simulink model "px4_control_system"  (R2023b)
settings: Solver=FixedStepAuto  StartTime=0.0  StopTime=inf  RelTol=1e-3  EnableMultiTasking=on
InitFcn:
  | prepare
values from neighbouring files (symbols this model uses):
  g = G_RPY18(x,p)    [CalculateLghn.m]
  m = 1    [CovarianceCheck.m]    (also in FL.m = in2(:,1); Fe1.m = in5(:,1); Fe1Fj.m = ct{4}; Fe1Gj.m = in5(:,1))
undefined symbols (not defined in the file or in its folder): AUX, color, dev, DiscIntNeverNeededParam, invC, J, led_mask, mode, pwm_output1
libraries: simulink x12, px4Sensorslib x4, px4uORBlib x2, px4lib x1
(part 2 of 2)

== matlab function px4_control_system/Subsystem/PX4 SD Card Logger1/SDCard_logger ==
  data: en input boolean; data input; logname parameter uint8; cacheflag parameter boolean; numRecs parameter uint32
%% PX4 SD Card Logger
% Note: All data needs to be of the same type (e.g. double)
% Header information format:
%           String "MWLOG"
%           Time/Date 4 bytes (time())
%           Number of Signals per record Logged 1 byte (256 max)
%           Data Type of Signals Logged  1 byte (1-10)
%           Number of bytes per record 2 bytes (65535 max)
% This does NOT include the number of data sets logged.
% i.e. The Reader is responsible for reading until EOF.
% Steve Kuznicki
% Copyright 2018 The MathWorks, Inc.

function SDCard_logger(en, data, logname, cacheflag, numRecs)

persistent fp isflushed isopen count  elem_size vect_size datastore timestore count_prev

if coder.target('Rtw')
    
    coder.cinclude('<stdio.h>');
    coder.cinclude('<time.h>');
    
    if coder.target('Rtw')
        coder.cinclude('<drivers/drv_hrt.h>');
    end
    
    if coder.target('Rtw')
        timestamp=coder.opaque('uint64_t');
        timestamp=coder.ceval('hrt_absolute_time');
    else
        timestamp = uint64(0);
    end
    
    if isempty(count)
        count = uint32(0);
        count_prev=count;
        fp = coder.opaque('FILE*', 'NULL');
        isflushed = false;
        if cacheflag == true
            datastore = zeros(numRecs*uint32(coder.const(numel(data))), 1, 'like', data);
            timestore=uint64(zeros(numRecs, 1));
        end
        
        [elsize, eltype] = get_elem_size(data);
        elem_size = coder.const(uint16(elsize));
        elem_type = coder.const(uint8(eltype));
        vect_size = coder.const(uint8(numel(data)));
        coder.ceval('printf',['OPENING file %s vect_size %d elem_size %d numRecs %d %c' uint8(0)], ...
            [logname,'.bin', int8(0)], uint32(vect_size), uint32(elem_size), uint32(numRecs), uint8(10));
        fp = coder.ceval('fopen', [logname,'.bin', int8(0)], ['wb', int8(0)]);
        isopen = true;
        
        % Write header information here
        % header token + version
        mlStrVer = 'MWLOG';
        coder.ceval('fwrite', coder.rref(mlStrVer), uint32(1), length(mlStrVer), fp);
        % date/time
        tm = uint32(0);
        tmptr = uint32(0);
        tm = coder.ceval('time',coder.wref(tmptr));
        coder.ceval('fwrite', coder.rref(tm), uint32(4), uint32(1), fp);
        % number of elements in each record
        coder.ceval('fwrite', coder.rref(vect_size), uint32(1), uint32(1), fp);
        % data type of the elements
        coder.ceval('fwrite', coder.rref(elem_type), uint32(1), uint32(1), fp);
        % size of each record in bytes
        recSize = elem_size * uint16(vect_size);
        coder.ceval('fwrite', coder.rref(recSize), uint32(2), uint32(1), fp);
    end
    
    
    if (en && (count < numRecs))
        
        if isopen == false
            % open file in append mode
            fp = coder.ceval('fopen', [logname,'.bin', int8(0)], ['ab', int8(0)]);
            isflushed = false;
            isopen = true;
            count_prev=count;
        end
        
        % cache data in memory or use fwrite
        if cacheflag == true
            addr = (count*uint32(vect_size))+1;
            for idx = 1:vect_size
                datastore(addr) = data(idx);
                addr = addr + 1;
            end
            timestore(count+uint32(1))=uint64(timestamp);
        else
            coder.ceval('fwrite', coder.rref(data), elem_size, vect_size, fp);
            if coder.target('Rtw')
                coder.ceval('fwrite', coder.rref(timestamp), uint32(8), uint32(1), fp);
            end
        end
        count = count + uint32(1);
        
    else
        if isopen == true
            if ~isflushed
                coder.ceval('printf',['CLOSING file. count = %d %c' uint8(0)], uint32(count), uint8(10));
                if cacheflag
                    for idx=count_prev+1:count
                        for idx2=(idx-1)*double(vect_size)+1:(idx-1)*double(vect_size)+double(vect_size)
                            coder.ceval('fwrite', coder.rref(datastore(idx2)), elem_size, uint32(1), fp);
                        end
                        coder.ceval('fwrite', coder.rref(timestore(idx)), uint32(8), uint32(1), fp);
                    end
                end
                coder.ceval('fflush', fp);
                isflushed = true;
            end
            coder.ceval('fclose', fp);
        end
        isopen = false;
    end
end

% return the size of the element in bytes
    function [elem_size, dtype] = get_elem_size(data)
        switch(class(data))
            case 'double'
                elem_size = 8;
                dtype = 1;
            case 'single'
                elem_size = 4;
                dtype = 2;
            case 'int32'
                elem_size = 4;
                dtype = 3;
            case 'uint32'
                elem_size = 4;
                dtype = 4;
            case 'int16'
                elem_size = 2;
                dtype = 5;
            case 'uint16'
                elem_size = 2;
                dtype = 6;
            case 'int8'
                elem_size = 1;
                dtype = 7;
            case 'uint8'
                elem_size = 1;
                dtype = 8;
            case 'logical'
                elem_size = 1;
                dtype = 9;
            case 'embedded.fi'
                nt = numerictype(data);
                elem_size = 2^ceil(log2(ceil(nt.WordLength / 8)));
                dtype = 10;
        end
        if ~isreal(data)
            elem_size = elem_size*2;
        end
        
        elem_size = uint16(elem_size);
        dtype = uint8(dtype);
    end
end

== matlab function px4_control_system/Control/MATLAB Function1 ==
  data: u input; y output
function y = ned2enu(u)
y = [u(2); u(1); -u(3)];

== matlab function px4_control_system/Subsystem/PX4 SD Card Logger2/SDCard_logger ==
  data: en input boolean; data input; logname parameter uint8; cacheflag parameter boolean; numRecs parameter uint32
%% PX4 SD Card Logger
% Note: All data needs to be of the same type (e.g. double)
% Header information format:
%           String "MWLOG"
%           Time/Date 4 bytes (time())
%           Number of Signals per record Logged 1 byte (256 max)
%           Data Type of Signals Logged  1 byte (1-10)
%           Number of bytes per record 2 bytes (65535 max)
% This does NOT include the number of data sets logged.
% i.e. The Reader is responsible for reading until EOF.
% Steve Kuznicki
% Copyright 2018 The MathWorks, Inc.

function SDCard_logger(en, data, logname, cacheflag, numRecs)

persistent fp isflushed isopen count  elem_size vect_size datastore timestore count_prev

if coder.target('Rtw')
    
    coder.cinclude('<stdio.h>');
    coder.cinclude('<time.h>');
    
    if coder.target('Rtw')
        coder.cinclude('<drivers/drv_hrt.h>');
    end
    
    if coder.target('Rtw')
        timestamp=coder.opaque('uint64_t');
        timestamp=coder.ceval('hrt_absolute_time');
    else
        timestamp = uint64(0);
    end
    
    if isempty(count)
        count = uint32(0);
        count_prev=count;
        fp = coder.opaque('FILE*', 'NULL');
        isflushed = false;
        if cacheflag == true
            datastore = zeros(numRecs*uint32(coder.const(numel(data))), 1, 'like', data);
            timestore=uint64(zeros(numRecs, 1));
        end
        
        [elsize, eltype] = get_elem_size(data);
        elem_size = coder.const(uint16(elsize));
        elem_type = coder.const(uint8(eltype));
        vect_size = coder.const(uint8(numel(data)));
        coder.ceval('printf',['OPENING file %s vect_size %d elem_size %d numRecs %d %c' uint8(0)], ...
            [logname,'.bin', int8(0)], uint32(vect_size), uint32(elem_size), uint32(numRecs), uint8(10));
        fp = coder.ceval('fopen', [logname,'.bin', int8(0)], ['wb', int8(0)]);
        isopen = true;
        
        % Write header information here
        % header token + version
        mlStrVer = 'MWLOG';
        coder.ceval('fwrite', coder.rref(mlStrVer), uint32(1), length(mlStrVer), fp);
        % date/time
        tm = uint32(0);
        tmptr = uint32(0);
        tm = coder.ceval('time',coder.wref(tmptr));
        coder.ceval('fwrite', coder.rref(tm), uint32(4), uint32(1), fp);
        % number of elements in each record
        coder.ceval('fwrite', coder.rref(vect_size), uint32(1), uint32(1), fp);
        % data type of the elements
        coder.ceval('fwrite', coder.rref(elem_type), uint32(1), uint32(1), fp);
        % size of each record in bytes
        recSize = elem_size * uint16(vect_size);
        coder.ceval('fwrite', coder.rref(recSize), uint32(2), uint32(1), fp);
    end
    
    
    if (en && (count < numRecs))
        
        if isopen == false
            % open file in append mode
            fp = coder.ceval('fopen', [logname,'.bin', int8(0)], ['ab', int8(0)]);
            isflushed = false;
            isopen = true;
            count_prev=count;
        end
        
        % cache data in memory or use fwrite
        if cacheflag == true
            addr = (count*uint32(vect_size))+1;
            for idx = 1:vect_size
                datastore(addr) = data(idx);
                addr = addr + 1;
            end
            timestore(count+uint32(1))=uint64(timestamp);
        else
            coder.ceval('fwrite', coder.rref(data), elem_size, vect_size, fp);
            if coder.target('Rtw')
                coder.ceval('fwrite', coder.rref(timestamp), uint32(8), uint32(1), fp);
            end
        end
        count = count + uint32(1);
        
    else
        if isopen == true
            if ~isflushed
                coder.ceval('printf',['CLOSING file. count = %d %c' uint8(0)], uint32(count), uint8(10));
                if cacheflag
                    for idx=count_prev+1:count
                        for idx2=(idx-1)*double(vect_size)+1:(idx-1)*double(vect_size)+double(vect_size)
                            coder.ceval('fwrite', coder.rref(datastore(idx2)), elem_size, uint32(1), fp);
                        end
                        coder.ceval('fwrite', coder.rref(timestore(idx)), uint32(8), uint32(1), fp);
                    end
                end
                coder.ceval('fflush', fp);
                isflushed = true;
            end
            coder.ceval('fclose', fp);
        end
        isopen = false;
    end
end

% return the size of the element in bytes
    function [elem_size, dtype] = get_elem_size(data)
        switch(class(data))
            case 'double'
                elem_size = 8;
                dtype = 1;
            case 'single'
                elem_size = 4;
                dtype = 2;
            case 'int32'
                elem_size = 4;
                dtype = 3;
            case 'uint32'
                elem_size = 4;
                dtype = 4;
            case 'int16'
                elem_size = 2;
                dtype = 5;
            case 'uint16'
                elem_size = 2;
                dtype = 6;
            case 'int8'
                elem_size = 1;
                dtype = 7;
            case 'uint8'
                elem_size = 1;
                dtype = 8;
            case 'logical'
                elem_size = 1;
                dtype = 9;
            case 'embedded.fi'
                nt = numerictype(data);
                elem_size = 2^ceil(log2(ceil(nt.WordLength / 8)));
                dtype = 10;
        end
        if ~isreal(data)
            elem_size = elem_size*2;
        end
        
        elem_size = uint16(elem_size);
        dtype = uint8(dtype);
    end
end

== matlab function px4_control_system/Subsystem/PX4 SD Card Logger3/SDCard_logger ==
  data: en input boolean; data input; logname parameter uint8; cacheflag parameter boolean; numRecs parameter uint32
%% PX4 SD Card Logger
% Note: All data needs to be of the same type (e.g. double)
% Header information format:
%           String "MWLOG"
%           Time/Date 4 bytes (time())
%           Number of Signals per record Logged 1 byte (256 max)
%           Data Type of Signals Logged  1 byte (1-10)
%           Number of bytes per record 2 bytes (65535 max)
% This does NOT include the number of data sets logged.
% i.e. The Reader is responsible for reading until EOF.
% Steve Kuznicki
% Copyright 2018 The MathWorks, Inc.

function SDCard_logger(en, data, logname, cacheflag, numRecs)

persistent fp isflushed isopen count  elem_size vect_size datastore timestore count_prev

if coder.target('Rtw')
    
    coder.cinclude('<stdio.h>');
    coder.cinclude('<time.h>');
    
    if coder.target('Rtw')
        coder.cinclude('<drivers/drv_hrt.h>');
    end
    
    if coder.target('Rtw')
        timestamp=coder.opaque('uint64_t');
        timestamp=coder.ceval('hrt_absolute_time');
    else
        timestamp = uint64(0);
    end
    
    if isempty(count)
        count = uint32(0);
        count_prev=count;
        fp = coder.opaque('FILE*', 'NULL');
        isflushed = false;
        if cacheflag == true
            datastore = zeros(numRecs*uint32(coder.const(numel(data))), 1, 'like', data);
            timestore=uint64(zeros(numRecs, 1));
        end
        
        [elsize, eltype] = get_elem_size(data);
        elem_size = coder.const(uint16(elsize));
        elem_type = coder.const(uint8(eltype));
        vect_size = coder.const(uint8(numel(data)));
        coder.ceval('printf',['OPENING file %s vect_size %d elem_size %d numRecs %d %c' uint8(0)], ...
            [logname,'.bin', int8(0)], uint32(vect_size), uint32(elem_size), uint32(numRecs), uint8(10));
        fp = coder.ceval('fopen', [logname,'.bin', int8(0)], ['wb', int8(0)]);
        isopen = true;
        
        % Write header information here
        % header token + version
        mlStrVer = 'MWLOG';
        coder.ceval('fwrite', coder.rref(mlStrVer), uint32(1), length(mlStrVer), fp);
        % date/time
        tm = uint32(0);
        tmptr = uint32(0);
        tm = coder.ceval('time',coder.wref(tmptr));
        coder.ceval('fwrite', coder.rref(tm), uint32(4), uint32(1), fp);
        % number of elements in each record
        coder.ceval('fwrite', coder.rref(vect_size), uint32(1), uint32(1), fp);
        % data type of the elements
        coder.ceval('fwrite', coder.rref(elem_type), uint32(1), uint32(1), fp);
        % size of each record in bytes
        recSize = elem_size * uint16(vect_size);
        coder.ceval('fwrite', coder.rref(recSize), uint32(2), uint32(1), fp);
    end
    
    
    if (en && (count < numRecs))
        
        if isopen == false
            % open file in append mode
            fp = coder.ceval('fopen', [logname,'.bin', int8(0)], ['ab', int8(0)]);
            isflushed = false;
            isopen = true;
            count_prev=count;
        end
        
        % cache data in memory or use fwrite
        if cacheflag == true
            addr = (count*uint32(vect_size))+1;
            for idx = 1:vect_size
                datastore(addr) = data(idx);
                addr = addr + 1;
            end
            timestore(count+uint32(1))=uint64(timestamp);
        else
            coder.ceval('fwrite', coder.rref(data), elem_size, vect_size, fp);
            if coder.target('Rtw')
                coder.ceval('fwrite', coder.rref(timestamp), uint32(8), uint32(1), fp);
            end
        end
        count = count + uint32(1);
        
    else
        if isopen == true
            if ~isflushed
                coder.ceval('printf',['CLOSING file. count = %d %c' uint8(0)], uint32(count), uint8(10));
                if cacheflag
                    for idx=count_prev+1:count
                        for idx2=(idx-1)*double(vect_size)+1:(idx-1)*double(vect_size)+double(vect_size)
                            coder.ceval('fwrite', coder.rref(datastore(idx2)), elem_size, uint32(1), fp);
                        end
                        coder.ceval('fwrite', coder.rref(timestore(idx)), uint32(8), uint32(1), fp);
                    end
                end
                coder.ceval('fflush', fp);
                isflushed = true;
            end
            coder.ceval('fclose', fp);
        end
        isopen = false;
    end
end

% return the size of the element in bytes
    function [elem_size, dtype] = get_elem_size(data)
        switch(class(data))
            case 'double'
                elem_size = 8;
                dtype = 1;
            case 'single'
                elem_size = 4;
                dtype = 2;
            case 'int32'
                elem_size = 4;
                dtype = 3;
            case 'uint32'
                elem_size = 4;
                dtype = 4;
            case 'int16'
                elem_size = 2;
                dtype = 5;
            case 'uint16'
                elem_size = 2;
                dtype = 6;
            case 'int8'
                elem_size = 1;
                dtype = 7;
            case 'uint8'
                elem_size = 1;
                dtype = 8;
            case 'logical'
                elem_size = 1;
                dtype = 9;
            case 'embedded.fi'
                nt = numerictype(data);
                elem_size = 2^ceil(log2(ceil(nt.WordLength / 8)));
                dtype = 10;
        end
        if ~isreal(data)
            elem_size = elem_size*2;
        end
        
        elem_size = uint16(elem_size);
        dtype = uint8(dtype);
    end
end

== matlab function px4_control_system/Control/MATLAB Function2 ==
  data: u input; y output
function y = limit_az(u)
y = u;
if(y<0)
    y=single(0);
end

== matlab function px4_control_system/Subsystem/PX4 SD Card Logger4/SDCard_logger ==
  data: en input boolean; data input; logname parameter uint8; cacheflag parameter boolean; numRecs parameter uint32
%% PX4 SD Card Logger
% Note: All data needs to be of the same type (e.g. double)
% Header information format:
%           String "MWLOG"
%           Time/Date 4 bytes (time())
%           Number of Signals per record Logged 1 byte (256 max)
%           Data Type of Signals Logged  1 byte (1-10)
%           Number of bytes per record 2 bytes (65535 max)
% This does NOT include the number of data sets logged.
% i.e. The Reader is responsible for reading until EOF.
% Steve Kuznicki
% Copyright 2018 The MathWorks, Inc.

function SDCard_logger(en, data, logname, cacheflag, numRecs)

persistent fp isflushed isopen count  elem_size vect_size datastore timestore count_prev

if coder.target('Rtw')
    
    coder.cinclude('<stdio.h>');
    coder.cinclude('<time.h>');
    
    if coder.target('Rtw')
        coder.cinclude('<drivers/drv_hrt.h>');
    end
    
    if coder.target('Rtw')
        timestamp=coder.opaque('uint64_t');
        timestamp=coder.ceval('hrt_absolute_time');
    else
        timestamp = uint64(0);
    end
    
    if isempty(count)
        count = uint32(0);
        count_prev=count;
        fp = coder.opaque('FILE*', 'NULL');
        isflushed = false;
        if cacheflag == true
            datastore = zeros(numRecs*uint32(coder.const(numel(data))), 1, 'like', data);
            timestore=uint64(zeros(numRecs, 1));
        end
        
        [elsize, eltype] = get_elem_size(data);
        elem_size = coder.const(uint16(elsize));
        elem_type = coder.const(uint8(eltype));
        vect_size = coder.const(uint8(numel(data)));
        coder.ceval('printf',['OPENING file %s vect_size %d elem_size %d numRecs %d %c' uint8(0)], ...
            [logname,'.bin', int8(0)], uint32(vect_size), uint32(elem_size), uint32(numRecs), uint8(10));
        fp = coder.ceval('fopen', [logname,'.bin', int8(0)], ['wb', int8(0)]);
        isopen = true;
        
        % Write header information here
        % header token + version
        mlStrVer = 'MWLOG';
        coder.ceval('fwrite', coder.rref(mlStrVer), uint32(1), length(mlStrVer), fp);
        % date/time
        tm = uint32(0);
        tmptr = uint32(0);
        tm = coder.ceval('time',coder.wref(tmptr));
        coder.ceval('fwrite', coder.rref(tm), uint32(4), uint32(1), fp);
        % number of elements in each record
        coder.ceval('fwrite', coder.rref(vect_size), uint32(1), uint32(1), fp);
        % data type of the elements
        coder.ceval('fwrite', coder.rref(elem_type), uint32(1), uint32(1), fp);
        % size of each record in bytes
        recSize = elem_size * uint16(vect_size);
        coder.ceval('fwrite', coder.rref(recSize), uint32(2), uint32(1), fp);
    end
    
    
    if (en && (count < numRecs))
        
        if isopen == false
            % open file in append mode
            fp = coder.ceval('fopen', [logname,'.bin', int8(0)], ['ab', int8(0)]);
            isflushed = false;
            isopen = true;
            count_prev=count;
        end
        
        % cache data in memory or use fwrite
        if cacheflag == true
            addr = (count*uint32(vect_size))+1;
            for idx = 1:vect_size
                datastore(addr) = data(idx);
                addr = addr + 1;
            end
            timestore(count+uint32(1))=uint64(timestamp);
        else
            coder.ceval('fwrite', coder.rref(data), elem_size, vect_size, fp);
            if coder.target('Rtw')
                coder.ceval('fwrite', coder.rref(timestamp), uint32(8), uint32(1), fp);
            end
        end
        count = count + uint32(1);
        
    else
        if isopen == true
            if ~isflushed
                coder.ceval('printf',['CLOSING file. count = %d %c' uint8(0)], uint32(count), uint8(10));
                if cacheflag
                    for idx=count_prev+1:count
                        for idx2=(idx-1)*double(vect_size)+1:(idx-1)*double(vect_size)+double(vect_size)
                            coder.ceval('fwrite', coder.rref(datastore(idx2)), elem_size, uint32(1), fp);
                        end
                        coder.ceval('fwrite', coder.rref(timestore(idx)), uint32(8), uint32(1), fp);
                    end
                end
                coder.ceval('fflush', fp);
                isflushed = true;
            end
            coder.ceval('fclose', fp);
        end
        isopen = false;
    end
end

% return the size of the element in bytes
    function [elem_size, dtype] = get_elem_size(data)
        switch(class(data))
            case 'double'
                elem_size = 8;
                dtype = 1;
            case 'single'
                elem_size = 4;
                dtype = 2;
            case 'int32'
                elem_size = 4;
                dtype = 3;
            case 'uint32'
                elem_size = 4;
                dtype = 4;
            case 'int16'
                elem_size = 2;
                dtype = 5;
            case 'uint16'
                elem_size = 2;
                dtype = 6;
            case 'int8'
                elem_size = 1;
                dtype = 7;
            case 'uint8'
                elem_size = 1;
                dtype = 8;
            case 'logical'
                elem_size = 1;
                dtype = 9;
            case 'embedded.fi'
                nt = numerictype(data);
                elem_size = 2^ceil(log2(ceil(nt.WordLength / 8)));
                dtype = 10;
        end
        if ~isreal(data)
            elem_size = elem_size*2;
        end
        
        elem_size = uint16(elem_size);
        dtype = uint8(dtype);
    end
end
